simulink model "uav"  (R2025b)
settings: Solver=VariableStepAuto  StartTime=0.0  StopTime=10.0  RelTol=1e-3
undefined symbols (not defined in the file or in its folder): CAMERA_NOISE_LEVEL, FOG_DENSITY_PERCENT, ILLUMINATION_LUX, OBS_X0, OBS_Y0, OBS_Z0, REQ_MIN_CLEARANCE, REQ_MIN_CONFIDENCE, UAV_X0, UAV_Y0, UAV_Z0
settings Model: Creator=lab  LastModifiedBy=lab

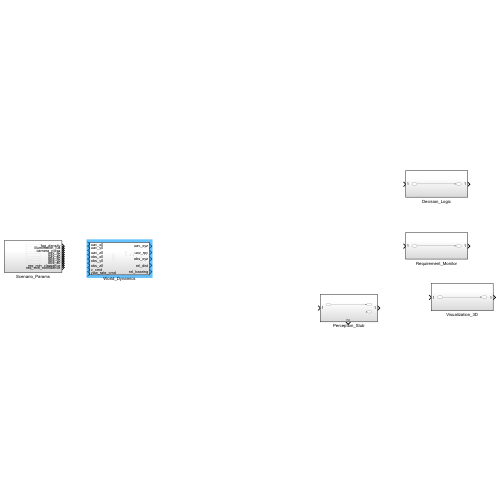
[thumbnail: Simulink's stored preview of the top-level diagram]
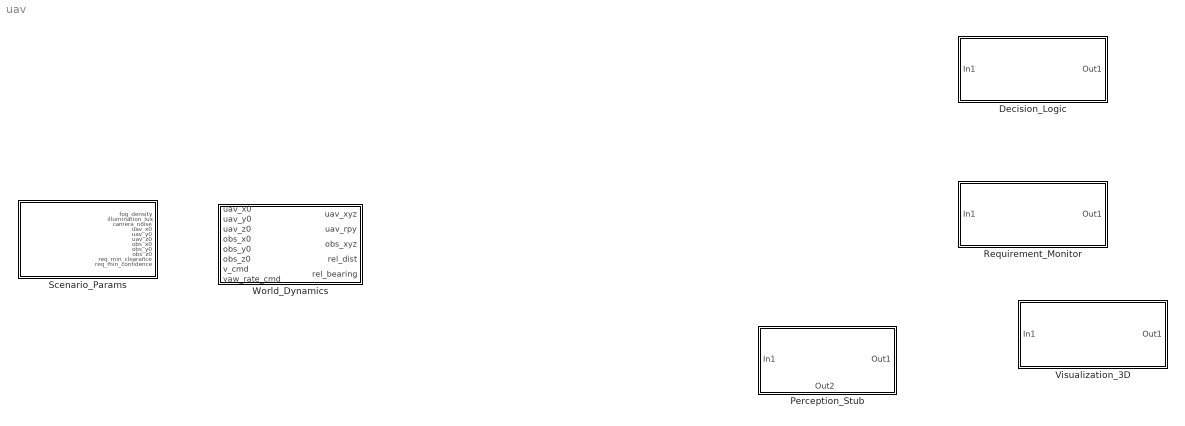
== system uav ==
  "Decision_Logic " : Subsystem
  Perception_Stub : Subsystem
      settings: PortSchema="{\"entries\":[{\"content\":{\"sides\":[{\"content\":{\"connectorIds\":[\"In1\"]},\"type\":\"ConnectorPlacement.EquallySpacedRectSide\",\"uuid\":\"57076dd3-6f9c-4de1-9ca8-63581b1c6389\"},{\"content\":{\"connectorIds\":[\"Out1\"],\"side\":\"RIGHT\"},\"type\":\"ConnectorPlacement.EquallySpacedRectSide\",\"uuid\":\"c400e5f3-d99a-4d44-bd94-c0d74ac21319\"},{\"content\":{\"side\":\"TOP\"},\"type\":\"ConnectorPlacement.EquallySpacedRectSide\",\"uuid\":\"30d8794d-4654-490d-946c-161f367a30ba\"},{\"content\":{\"connectorIds\":[\"Out2\"],\"side\":\"BOTTOM\"},\"type\":\"ConnectorPlacement.EquallySpacedRectSide\",\"uuid\":\"2b9a873c-0cfc-4b93-9e4e-4aa2e22d06c3\"}]},\"type\":\"ConnectorPlacement.EquallySpacedConnector\",\"uuid\":\"81d34601-1143-492d-bab0-7bd999da64e3\"}],\"packageUris\":[\"http://schema.mathworks.com/mf0/Connector/R2020b\"],\"version\":\"1.0\"}"
  Requirement_Monitor : Subsystem
  Scenario_Params : Subsystem
  Visualization_3D : Subsystem
  World_Dynamics : Subsystem

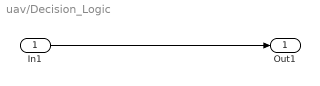
== system uav/Decision_Logic  ==
  In1 : Inport
  Out1 : Outport
  wires:
  In1/1 -> Out1/1

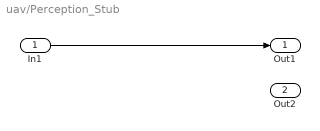
== system uav/Perception_Stub ==
  In1 : Inport
  Out1 : Outport
  Out2 : Outport  Port=2
  wires:
  In1/1 -> Out1/1

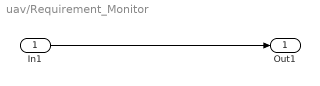
== system uav/Requirement_Monitor ==
  In1 : Inport
  Out1 : Outport
  wires:
  In1/1 -> Out1/1

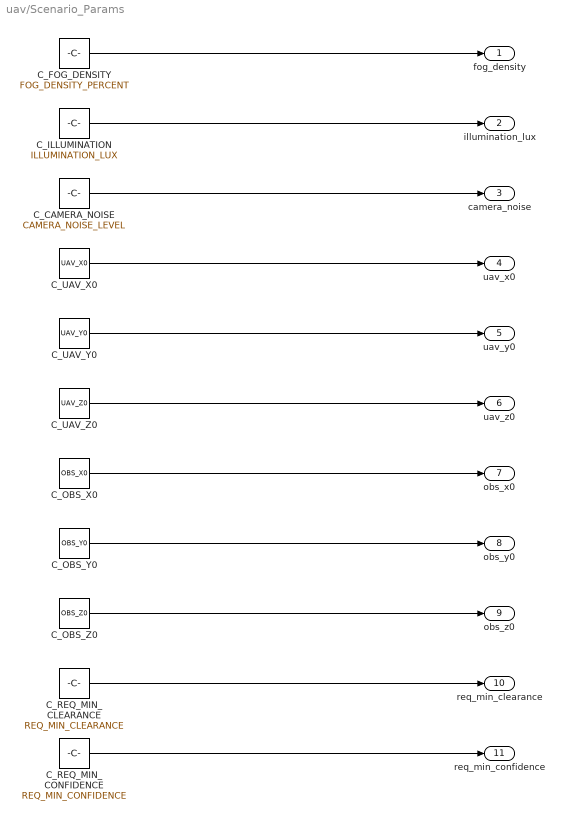
== system uav/Scenario_Params ==
  C_CAMERA_NOISE : Constant  Value=CAMERA_NOISE_LEVEL
  C_FOG_DENSITY : Constant  Value=FOG_DENSITY_PERCENT
  C_ILLUMINATION : Constant  Value=ILLUMINATION_LUX
  C_OBS_X0 : Constant  Value=OBS_X0
  C_OBS_Y0 : Constant  Value=OBS_Y0
  C_OBS_Z0 : Constant  Value=OBS_Z0
  C_REQ_MIN_CLEARANCE : Constant  Value=REQ_MIN_CLEARANCE
  C_REQ_MIN_CONFIDENCE : Constant  Value=REQ_MIN_CONFIDENCE
  C_UAV_X0 : Constant  Value=UAV_X0
  C_UAV_Y0 : Constant  Value=UAV_Y0
  C_UAV_Z0 : Constant  Value=UAV_Z0
  fog_density : Outport
  illumination_lux : Outport  Port=2
  camera_noise : Outport  Port=3
  uav_x0 : Outport  Port=4
  uav_y0 : Outport  Port=5
  uav_z0 : Outport  Port=6
  obs_x0 : Outport  Port=7
  obs_y0 : Outport  Port=8
  obs_z0 : Outport  Port=9
  req_min_clearance : Outport  Port=10
  req_min_confidence : Outport  Port=11
  wires:
  C_FOG_DENSITY/1 -> fog_density/1
  C_ILLUMINATION/1 -> illumination_lux/1
  C_CAMERA_NOISE/1 -> camera_noise/1
  C_UAV_X0/1 -> uav_x0/1
  C_UAV_Y0/1 -> uav_y0/1
  C_UAV_Z0/1 -> uav_z0/1
  C_OBS_X0/1 -> obs_x0/1
  C_OBS_Y0/1 -> obs_y0/1
  C_OBS_Z0/1 -> obs_z0/1
  C_REQ_MIN_CLEARANCE/1 -> req_min_clearance/1
  C_REQ_MIN_CONFIDENCE/1 -> req_min_confidence/1

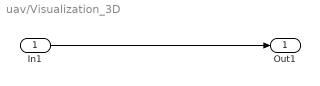
== system uav/Visualization_3D ==
  In1 : Inport
  Out1 : Outport
  wires:
  In1/1 -> Out1/1

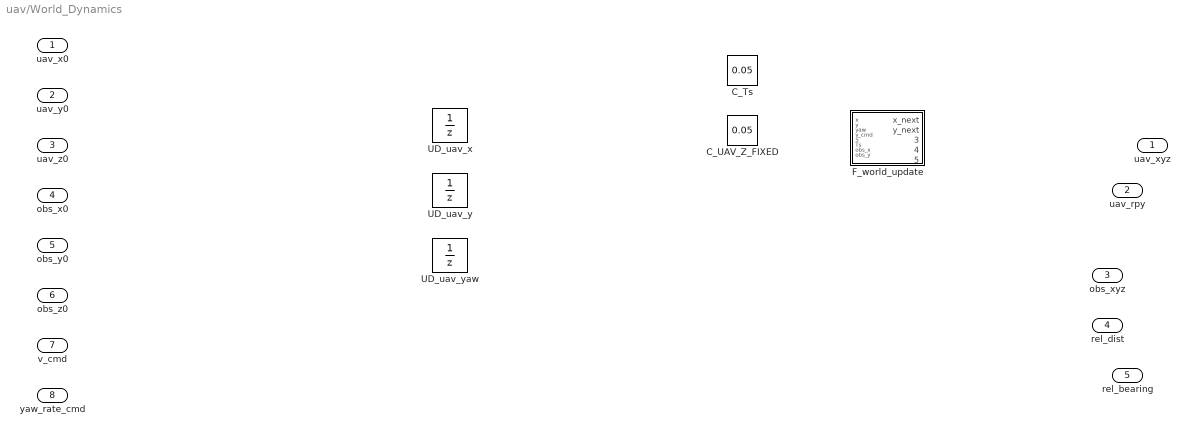
== system uav/World_Dynamics ==
  uav_x0 : Inport
  uav_y0 : Inport  Port=2
  uav_z0 : Inport  Port=3
  obs_x0 : Inport  Port=4
  obs_y0 : Inport  Port=5
  obs_z0 : Inport  Port=6
  v_cmd : Inport  Port=7
  yaw_rate_cmd : Inport  Port=8
  C_Ts : Constant  Value=0.05
  C_UAV_Z_FIXED : Constant  Value=0.05
  F_world_update : MATLAB Function  TreatAsAtomicUnit=on
  UD_uav_x : UnitDelay  SampleTime=-1  HasFrameUpgradeWarning=on
  UD_uav_y : UnitDelay  SampleTime=-1  HasFrameUpgradeWarning=on
  UD_uav_yaw : UnitDelay  SampleTime=-1  HasFrameUpgradeWarning=on
  uav_xyz : Outport
  uav_rpy : Outport  Port=2
  obs_xyz : Outport  Port=3
  rel_dist : Outport  Port=4
  rel_bearing : Outport  Port=5

== matlab function uav/World_Dynamics/F_world_update ==
  data: x input; x_next output; y input; yaw input; v_cmd input; yaw_rate_cmd input; Ts input; obs_x input; obs_y input; y_next output; yaw_next output; rel_dist output; rel_bearing output
function [x_next, y_next, yaw_next, rel_dist, rel_bearing] = ...
    F_world_update(x, y, yaw, v_cmd, yaw_rate_cmd, Ts, obs_x, obs_y)

x_next = x + Ts * v_cmd * cos(yaw);
y_next = y + Ts * v_cmd * sin(yaw);
yaw_next = yaw + Ts * yaw_rate_cmd;

dx = obs_x - x_next;
dy = obs_y - y_next;

rel_dist = sqrt(dx^2 + dy^2);
rel_bearing = atan2(dy, dx) - yaw_next;
end
